simulink library "experiment_lib"  (Simulink 7.1)
values from neighbouring files (symbols this model uses):
  denPQ = [1 -0.999371878799]    [Pau_Pol_6_Nodes_4_Perd_0_TxRate_0.01.mat]
  LL = [0.000782892151765 0.000588394714514 0.000709966836418 0.00082261967749]    [Pau_Pol_6_Nodes_4_Perd_0_TxRate_0.01.mat]    (also in llencadora_sim.m = minLL+(maxLL-minLL)*rand(1,num_loads))
  Lline = [1.0827664502e-05 1.06430432216e-05 1.0255354423e-05 1.05299829153e-05]    [Pau_Pol_6_Nodes_4_Perd_0_TxRate_0.01.mat]    (also in llencadora_sim.m = minLline+(maxLline-minLline)*rand(1,num_lines))
  Lv = 1.28e-05    [Pau_Pol_6_Nodes_4_Perd_0_TxRate_0.01.mat]    (also in llencadora_sim.m = Lvm(nodes); processor.m = data.Lv)
  m = 1e-05    [Pau_Pol_6_Nodes_4_Perd_0_TxRate_0.01.mat]    (also in llencadora_sim.m; processor.m = data.m)
  mp = 5e-07    [Pau_Pol_6_Nodes_4_Perd_0_TxRate_0.01.mat]    (also in llencadora_sim.m = mpm(nodes); processor.m = data.mp)
  n = 0.0001    [Pau_Pol_6_Nodes_4_Perd_0_TxRate_0.01.mat]    (also in llencadora_sim.m; processor.m = data.n)
  numPQ = [0.000314060600312 0.000314060600312]    [Pau_Pol_6_Nodes_4_Perd_0_TxRate_0.01.mat]
  RL = [0.345490722943 0.282580500651 0.390474448437 0.324054882207]    [Pau_Pol_6_Nodes_4_Perd_0_TxRate_0.01.mat]    (also in llencadora_sim.m = minRL+(maxRL-minRL)*rand(1,num_loads))
  Rline = [0.00149363403679 0.00820725625814 0.00655593060546 0.00272568602759]    [Pau_Pol_6_Nodes_4_Perd_0_TxRate_0.01.mat]    (also in llencadora_sim.m = minRline+(maxRline-minRline)*rand(1,num_lines))
  tr = 0.01    [Pau_Pol_6_Nodes_4_Perd_0_TxRate_0.01.mat]    (also in llencadora_sim.m = 10)
  ts = 0.0001    [Pau_Pol_6_Nodes_4_Perd_0_TxRate_0.01.mat]    (also in dintegral_w_code.m; llencadora_sim.m; processor.m = data.ts)
  Vn = 325.269119346    [Pau_Pol_6_Nodes_4_Perd_0_TxRate_0.01.mat]    (also in llencadora_sim.m = 230*sqrt(2); processor.m = data.Vn)
  wo = 314.159265359    [Pau_Pol_6_Nodes_4_Perd_0_TxRate_0.01.mat]    (also in llencadora_sim.m; processor.m = data.wo)
undefined symbols (not defined in the file or in its folder): CL
libraries: powerlib x24, truetime x2
settings Model: Creator=SEPIC  LastModifiedBy=SEPIC

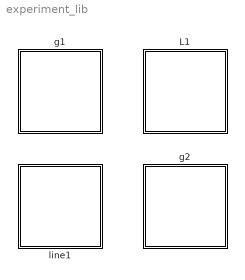
== system experiment_lib ==
  L1 : Subsystem  Orientation=down  mask{a=1}
      mask Display: disp(['Load' num2str(a)])
  g1 : Subsystem  Orientation=down  mask{a=1}
      mask Display: disp(['Gen' num2str(a)]);port_label('PMC',1,'a')
  g2 : Subsystem  Orientation=down  mask{a=1}
      mask Display: disp(['GenCom' num2str(a)]);port_label('PMC',1,'a')
  line1 : Subsystem  Orientation=left  mask{a=1}
      mask Display: disp(['Line' num2str(a)]);

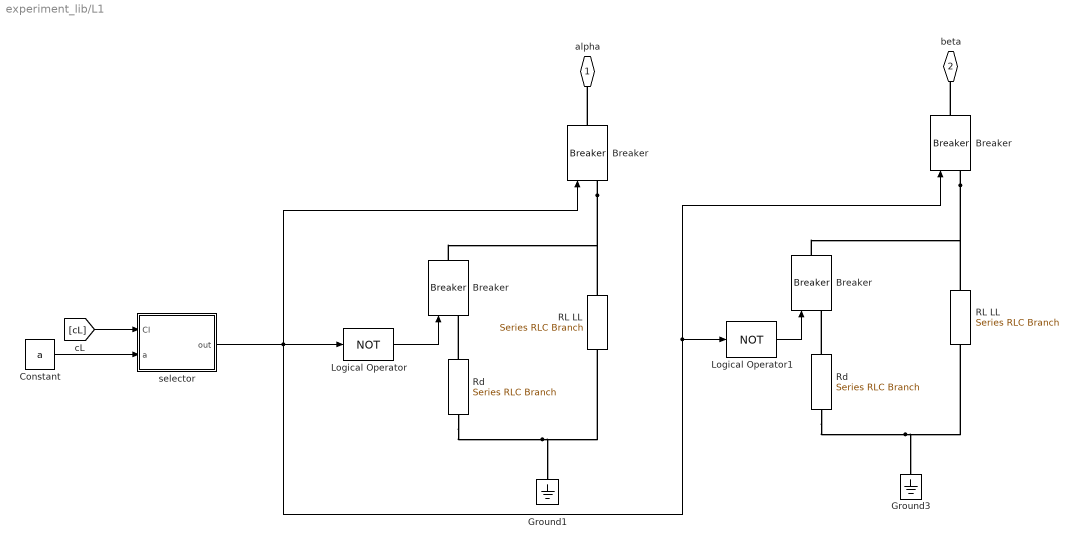
== system experiment_lib/L1 ==
  "  Rd" : powerlib/Elements/Series RLC Branch  Orientation=down  DialogController=POWERSYS.PowerSysDialog  PhysicalDomain=powersysdomain  SubClassName=unknown  LeftPortType=p1  RightPortType=p1  LConnTagsString=__new0  RConnTagsString=__new0  BranchType=R  Resistance=1  Inductance=1.0  SetiL0=off  InitialCurrent=0  Capacitance=CL  Setx0=off  InitialVoltage=0  Measurements=None
  "  Rd  " : powerlib/Elements/Series RLC Branch  Orientation=down  DialogController=POWERSYS.PowerSysDialog  PhysicalDomain=powersysdomain  SubClassName=unknown  LeftPortType=p1  RightPortType=p1  LConnTagsString=__new0  RConnTagsString=__new0  BranchType=R  Resistance=1  Inductance=1.0  SetiL0=off  InitialCurrent=0  Capacitance=CL  Setx0=off  InitialVoltage=0  Measurements=None
  Breaker : powerlib/Elements/Breaker  Orientation=up  DialogController=POWERSYS.PowerSysDialog  SystemSampleTime=-1  BreakerResistance=10e-6  InitialState=0  SnubberResistance=1e6  SnubberCapacitance=inf  SwitchingTimes="[ 1/60  5/60 ]"  External=on  Measurements=None  MoreParameters=off  NoBreakLoop=off
  "Breaker " : powerlib/Elements/Breaker  Orientation=up  DialogController=POWERSYS.PowerSysDialog  SystemSampleTime=-1  BreakerResistance=10e-6  InitialState=0  SnubberResistance=1e6  SnubberCapacitance=inf  SwitchingTimes="[ 1/60  5/60 ]"  External=on  Measurements=None  MoreParameters=off  NoBreakLoop=off
  "Breaker   " : powerlib/Elements/Breaker  Orientation=up  DialogController=POWERSYS.PowerSysDialog  SystemSampleTime=-1  BreakerResistance=10e-6  InitialState=0  SnubberResistance=1e6  SnubberCapacitance=inf  SwitchingTimes="[ 1/60  5/60 ]"  External=on  Measurements=None  MoreParameters=off  NoBreakLoop=off
  "Breaker      " : powerlib/Elements/Breaker  Orientation=up  DialogController=POWERSYS.PowerSysDialog  SystemSampleTime=-1  BreakerResistance=10e-6  InitialState=0  SnubberResistance=1e6  SnubberCapacitance=inf  SwitchingTimes="[ 1/60  5/60 ]"  External=on  Measurements=None  MoreParameters=off  NoBreakLoop=off
  Constant : Constant  Value=a  OutDataType=sfix(16)  OutScaling=2^0
  Ground1 : powerlib/Elements/Ground  Orientation=down  DialogController=POWERSYS.PowerSysDialog  PhysicalDomain=powersysdomain  SubClassName=unknown  LeftPortType=p1  RightPortType=p1  LConnTagsString=a
  Ground3 : powerlib/Elements/Ground  Orientation=down  DialogController=POWERSYS.PowerSysDialog  PhysicalDomain=powersysdomain  SubClassName=unknown  LeftPortType=p1  RightPortType=p1  LConnTagsString=a
  Logical Operator : Logic  Operator=NOT  AllPortsSameDT=off  OutDataTypeMode=boolean  OutDataTypeStr=boolean
  Logical Operator1 : Logic  Operator=NOT  AllPortsSameDT=off  OutDataTypeMode=boolean  OutDataTypeStr=boolean
  RL LL : powerlib/Elements/Series RLC Branch  Orientation=down  DialogController=POWERSYS.PowerSysDialog  PhysicalDomain=powersysdomain  SubClassName=unknown  LeftPortType=p1  RightPortType=p1  LConnTagsString=__new0  RConnTagsString=__new0  BranchType=RL  Resistance=RL(a)  Inductance=LL(a)  SetiL0=off  InitialCurrent=0  Capacitance=CL  Setx0=off  InitialVoltage=0  Measurements=None
  "RL LL   " : powerlib/Elements/Series RLC Branch  Orientation=down  DialogController=POWERSYS.PowerSysDialog  PhysicalDomain=powersysdomain  SubClassName=unknown  LeftPortType=p1  RightPortType=p1  LConnTagsString=__new0  RConnTagsString=__new0  BranchType=RL  Resistance=RL(a)  Inductance=LL(a)  SetiL0=off  InitialCurrent=0  Capacitance=CL  Setx0=off  InitialVoltage=0  Measurements=None
  selector : Stateflow chart  TreatAsAtomicUnit=on
  "alpha " : PMIOPort  Orientation=down  Port=1  Side=Left
  beta : PMIOPort  Orientation=down  Port=2  Side=Left
  wires:
  Logical Operator/1 -> Breaker/1
  selector/1(out) -> Logical Operator/1, "Breaker      "/1, Logical Operator1/1, "Breaker   "/1
  Logical Operator1/1 -> "Breaker "/1
  [cL] -> selector/1(Cl)
  Constant/1 -> selector/2(a)
  connections:
  "Breaker      "/LConn1 -- Breaker/RConn1 -- RL LL/LConn1
  "  Rd"/RConn1 -- RL LL/RConn1 -- Ground1/LConn1
  "  Rd"/LConn1 -- Breaker/LConn1
  "Breaker      "/RConn1 -- "alpha "/RConn1
  "Breaker   "/LConn1 -- "RL LL   "/LConn1 -- "Breaker "/RConn1
  "  Rd  "/RConn1 -- Ground3/LConn1 -- "RL LL   "/RConn1
  "  Rd  "/LConn1 -- "Breaker "/LConn1
  "Breaker   "/RConn1 -- beta/RConn1

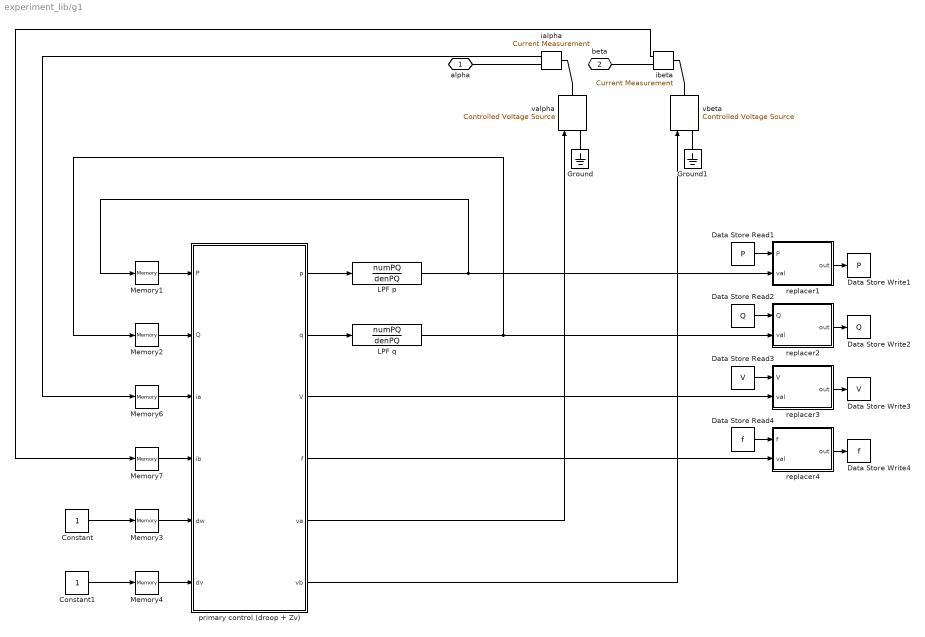
== system experiment_lib/g1 ==
  Constant : Constant  OutDataType=sfix(16)  OutScaling=2^0
  Constant1 : Constant  OutDataType=sfix(16)  OutScaling=2^0
  Data Store Read1 : DataStoreRead  DataStoreName=P  SampleTime=0
  Data Store Read2 : DataStoreRead  DataStoreName=Q  SampleTime=0
  Data Store Read3 : DataStoreRead  DataStoreName=V  SampleTime=0
  Data Store Read4 : DataStoreRead  DataStoreName=f  SampleTime=0
  Data Store Write1 : DataStoreWrite  DataStoreName=P  SampleTime=-1
  Data Store Write2 : DataStoreWrite  DataStoreName=Q  SampleTime=-1
  Data Store Write3 : DataStoreWrite  DataStoreName=V  SampleTime=-1
  Data Store Write4 : DataStoreWrite  DataStoreName=f  SampleTime=-1
  Ground : powerlib/Elements/Ground  Orientation=down  DialogController=POWERSYS.PowerSysDialog  PhysicalDomain=powersysdomain  SubClassName=unknown  LeftPortType=p1  RightPortType=p1  LConnTagsString=a
  Ground1 : powerlib/Elements/Ground  Orientation=down  DialogController=POWERSYS.PowerSysDialog  PhysicalDomain=powersysdomain  SubClassName=unknown  LeftPortType=p1  RightPortType=p1  LConnTagsString=a
  LPF p : DiscreteTransferFcn  Numerator=numPQ  Denominator=denPQ  SampleTime=ts
  LPF q : DiscreteTransferFcn  Numerator=numPQ  Denominator=denPQ  SampleTime=ts
  Memory{1..4,6..7} (6 alike) : Memory
  ialpha : powerlib/Measurements/Current Measurement  Orientation=left  DialogController=POWERSYS.PowerSysDialog  SystemSampleTime=-1  PhasorSimulation=off  OutputType=Complex  PSBequivalent=0
  ibeta : powerlib/Measurements/Current Measurement  Orientation=left  DialogController=POWERSYS.PowerSysDialog  SystemSampleTime=-1  PhasorSimulation=off  OutputType=Complex  PSBequivalent=0
  primary control (droop + Zv) : Stateflow chart  TreatAsAtomicUnit=on
  replacer1 : Stateflow chart  TreatAsAtomicUnit=on
  replacer2 : Stateflow chart  TreatAsAtomicUnit=on
  replacer3 : Stateflow chart  TreatAsAtomicUnit=on
  replacer4 : Stateflow chart  TreatAsAtomicUnit=on
  valpha : powerlib/Electrical Sources/Controlled Voltage Source  Orientation=up  DialogController=POWERSYS.PowerSysDialog  SystemSampleTime=-1  Initialize=on  Source_Type=AC  Amplitude=0  Phase=0  Frequency=0  Measurements=None
  vbeta : powerlib/Electrical Sources/Controlled Voltage Source  Orientation=up  DialogController=POWERSYS.PowerSysDialog  SystemSampleTime=-1  Initialize=on  Source_Type=AC  Amplitude=0  Phase=0  Frequency=0  Measurements=None
  alpha : PMIOPort  Port=1  Side=Left
  beta : PMIOPort  Port=2  Side=Left
  wires:
  ibeta/1 -> Memory7/1
  ialpha/1 -> Memory6/1
  LPF p/1 -> Memory1/1, replacer1/2(val)
  LPF q/1 -> Memory2/1, replacer2/2(val)
  primary control (droop + Zv)/1(p) -> LPF p/1
  primary control (droop + Zv)/2(q) -> LPF q/1
  primary control (droop + Zv)/4(f) -> replacer4/2(val)
  primary control (droop + Zv)/3(V) -> replacer3/2(val)
  Memory6/1 -> primary control (droop + Zv)/3(ia)
  Memory7/1 -> primary control (droop + Zv)/4(ib)
  Memory1/1 -> primary control (droop + Zv)/1(P)
  Memory2/1 -> primary control (droop + Zv)/2(Q)
  Memory3/1 -> primary control (droop + Zv)/5(dw)
  Memory4/1 -> primary control (droop + Zv)/6(dv)
  primary control (droop + Zv)/5(va) -> valpha/1
  primary control (droop + Zv)/6(vb) -> vbeta/1
  Constant/1 -> Memory3/1
  Constant1/1 -> Memory4/1
  replacer1/1(out) -> Data Store Write1/1
  replacer2/1(out) -> Data Store Write2/1
  Data Store Read2/1 -> replacer2/1(Q)
  replacer3/1(out) -> Data Store Write3/1
  Data Store Read3/1 -> replacer3/1(V)
  Data Store Read1/1 -> replacer1/1(P)
  replacer4/1(out) -> Data Store Write4/1
  Data Store Read4/1 -> replacer4/1(f)
  connections:
  Ground1/LConn1 -- vbeta/LConn1
  valpha/RConn1 -- ialpha/LConn1
  beta/RConn1 -- ibeta/RConn1
  vbeta/RConn1 -- ibeta/LConn1
  Ground/LConn1 -- valpha/LConn1
  alpha/RConn1 -- ialpha/RConn1

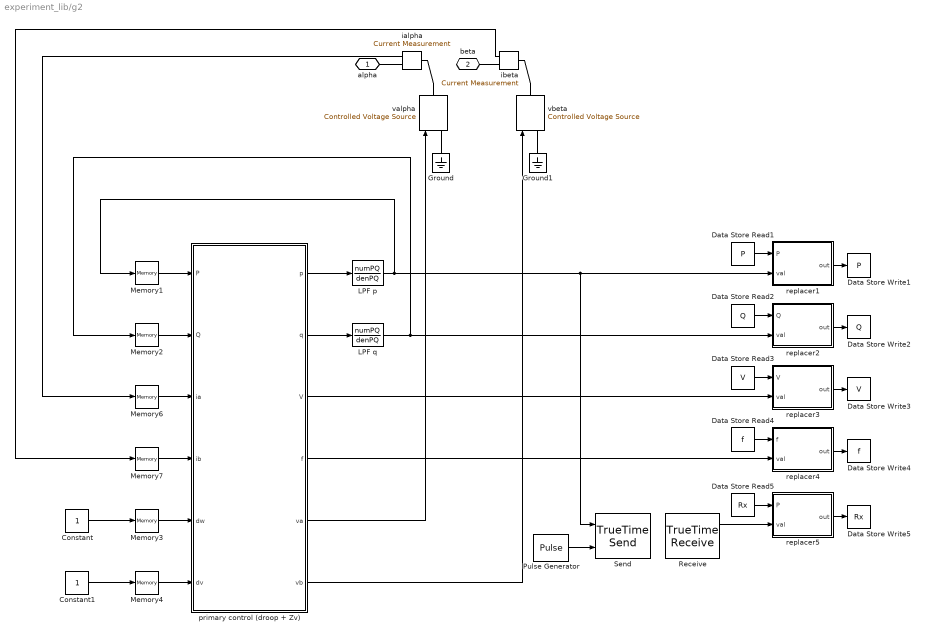
== system experiment_lib/g2 ==
  Constant : Constant  OutDataType=sfix(16)  OutScaling=2^0
  Constant1 : Constant  OutDataType=sfix(16)  OutScaling=2^0
  Data Store Read1 : DataStoreRead  DataStoreName=P  SampleTime=0
  Data Store Read2 : DataStoreRead  DataStoreName=Q  SampleTime=0
  Data Store Read3 : DataStoreRead  DataStoreName=V  SampleTime=0
  Data Store Read4 : DataStoreRead  DataStoreName=f  SampleTime=0
  Data Store Read5 : DataStoreRead  DataStoreName=Rx  SampleTime=0
  Data Store Write1 : DataStoreWrite  DataStoreName=P  SampleTime=-1
  Data Store Write2 : DataStoreWrite  DataStoreName=Q  SampleTime=-1
  Data Store Write3 : DataStoreWrite  DataStoreName=V  SampleTime=-1
  Data Store Write4 : DataStoreWrite  DataStoreName=f  SampleTime=-1
  Data Store Write5 : DataStoreWrite  DataStoreName=Rx  SampleTime=-1
  Ground : powerlib/Elements/Ground  Orientation=down  DialogController=POWERSYS.PowerSysDialog  PhysicalDomain=powersysdomain  SubClassName=unknown  LeftPortType=p1  RightPortType=p1  LConnTagsString=a
  Ground1 : powerlib/Elements/Ground  Orientation=down  DialogController=POWERSYS.PowerSysDialog  PhysicalDomain=powersysdomain  SubClassName=unknown  LeftPortType=p1  RightPortType=p1  LConnTagsString=a
  LPF p : DiscreteTransferFcn  Numerator=numPQ  Denominator=denPQ  SampleTime=ts
  LPF q : DiscreteTransferFcn  Numerator=numPQ  Denominator=denPQ  SampleTime=ts
  Memory{1..4,6..7} (6 alike) : Memory
  Pulse Generator : DiscretePulseGenerator  PulseType=Time based  Period=tr  PulseWidth=50
  Receive : truetime/TrueTime Receive  SystemSampleTime=-1  nwnbr=1  receiver=a  outdim=1  triggeroutput=off  senderoutput=on  lengthoutput=off  priorityoutput=off  timestampoutput=off  signalpoweroutput=off  msgIDoutput=off
  Send : truetime/TrueTime Send  SystemSampleTime=-1  trigger=rising  nwnbr=1  sender=a  indim=1  recsource=internal  receiver=0  lengthsource=internal  length=80  priosource=internal  prio=2  msgIDsource=internal  msgID=0  dynamicSegment=dynamic
  ialpha : powerlib/Measurements/Current Measurement  Orientation=left  DialogController=POWERSYS.PowerSysDialog  SystemSampleTime=-1  PhasorSimulation=off  OutputType=Complex  PSBequivalent=0
  ibeta : powerlib/Measurements/Current Measurement  Orientation=left  DialogController=POWERSYS.PowerSysDialog  SystemSampleTime=-1  PhasorSimulation=off  OutputType=Complex  PSBequivalent=0
  primary control (droop + Zv) : Stateflow chart  TreatAsAtomicUnit=on
  replacer1 : Stateflow chart  TreatAsAtomicUnit=on
  replacer2 : Stateflow chart  TreatAsAtomicUnit=on
  replacer3 : Stateflow chart  TreatAsAtomicUnit=on
  replacer4 : Stateflow chart  TreatAsAtomicUnit=on
  replacer5 : Stateflow chart  TreatAsAtomicUnit=on
  valpha : powerlib/Electrical Sources/Controlled Voltage Source  Orientation=up  DialogController=POWERSYS.PowerSysDialog  SystemSampleTime=-1  Initialize=on  Source_Type=AC  Amplitude=0  Phase=0  Frequency=0  Measurements=None
  vbeta : powerlib/Electrical Sources/Controlled Voltage Source  Orientation=up  DialogController=POWERSYS.PowerSysDialog  SystemSampleTime=-1  Initialize=on  Source_Type=AC  Amplitude=0  Phase=0  Frequency=0  Measurements=None
  alpha : PMIOPort  Port=1  Side=Left
  beta : PMIOPort  Port=2  Side=Left
  wires:
  Data Store Read4/1 -> replacer4/1(f)
  replacer4/1(out) -> Data Store Write4/1
  Data Store Read1/1 -> replacer1/1(P)
  Data Store Read3/1 -> replacer3/1(V)
  replacer3/1(out) -> Data Store Write3/1
  Data Store Read2/1 -> replacer2/1(Q)
  replacer2/1(out) -> Data Store Write2/1
  replacer1/1(out) -> Data Store Write1/1
  Constant1/1 -> Memory4/1
  Constant/1 -> Memory3/1
  primary control (droop + Zv)/6(vb) -> vbeta/1
  primary control (droop + Zv)/5(va) -> valpha/1
  Memory4/1 -> primary control (droop + Zv)/6(dv)
  Memory3/1 -> primary control (droop + Zv)/5(dw)
  Memory2/1 -> primary control (droop + Zv)/2(Q)
  Memory1/1 -> primary control (droop + Zv)/1(P)
  Memory7/1 -> primary control (droop + Zv)/4(ib)
  Memory6/1 -> primary control (droop + Zv)/3(ia)
  primary control (droop + Zv)/3(V) -> replacer3/2(val)
  primary control (droop + Zv)/4(f) -> replacer4/2(val)
  primary control (droop + Zv)/2(q) -> LPF q/1
  primary control (droop + Zv)/1(p) -> LPF p/1
  LPF q/1 -> replacer2/2(val), Memory2/1
  LPF p/1 -> Memory1/1, replacer1/2(val), Send/1
  ialpha/1 -> Memory6/1
  ibeta/1 -> Memory7/1
  Pulse Generator/1 -> Send/2
  Data Store Read5/1 -> replacer5/1(P)
  replacer5/1(out) -> Data Store Write5/1
  Receive/1 -> replacer5/2(val)
  connections:
  alpha/RConn1 -- ialpha/RConn1
  Ground/LConn1 -- valpha/LConn1
  vbeta/RConn1 -- ibeta/LConn1
  beta/RConn1 -- ibeta/RConn1
  valpha/RConn1 -- ialpha/LConn1
  Ground1/LConn1 -- vbeta/LConn1

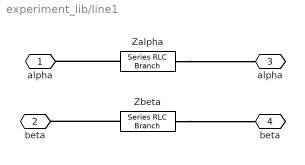
== system experiment_lib/line1 ==
  Zalpha : powerlib/Elements/Series RLC Branch  Orientation=left  DialogController=POWERSYS.PowerSysDialog  PhysicalDomain=powersysdomain  SubClassName=unknown  LeftPortType=p1  RightPortType=p1  LConnTagsString=__new0  RConnTagsString=__new0  BranchType=RL  Resistance=Rline(a)  Inductance=Lline(a)  SetiL0=off  InitialCurrent=0  Capacitance=CL  Setx0=off  InitialVoltage=0  Measurements=None
  Zbeta : powerlib/Elements/Series RLC Branch  Orientation=left  DialogController=POWERSYS.PowerSysDialog  PhysicalDomain=powersysdomain  SubClassName=unknown  LeftPortType=p1  RightPortType=p1  LConnTagsString=__new0  RConnTagsString=__new0  BranchType=RL  Resistance=Rline(a)  Inductance=Lline(a)  SetiL0=off  InitialCurrent=0  Capacitance=CL  Setx0=off  InitialVoltage=0  Measurements=None
  alpha : PMIOPort  Port=1  Side=Left
  "beta " : PMIOPort  Port=2  Side=Left
  "alpha " : PMIOPort  Orientation=left  Port=3  Side=Right
  "beta   " : PMIOPort  Orientation=left  Port=4  Side=Right
  connections:
  Zbeta/RConn1 -- "beta "/RConn1
  Zbeta/LConn1 -- "beta   "/RConn1
  Zalpha/RConn1 -- alpha/RConn1
  Zalpha/LConn1 -- "alpha "/RConn1

== matlab function g1/replacer1 ==
  data: P input double; out output double; val input double; a parameter double
function out  = fcn2(P,val,a)
out=P;
out(a)=val;

== matlab function g1/replacer2 ==
  data: Q input double; out output double; val input double; a parameter double
function out  = fcn2(Q,val,a)
out=Q;
out(a)=val;

== matlab function g1/replacer3 ==
  data: V input double; out output double; val input double; a parameter double
function out  = fcn2(V,val,a)
out=V;
out(a)=val;

== matlab function L1/selector ==
  data: Cl input double; out output double; a input double
function out  = fcn2(Cl,a)
out=Cl(a);

== matlab function g1/replacer4 ==
  data: f input double; out output double; val input double; a parameter double
function out  = fcn2(f,val,a)
out=f;
out(a)=val;

== matlab function g2/primary control (droop + Zv) ==
  settings: updateMethod=DISCRETE  sampleTime=ts
  data: P input double; Q input double; ia input double size=1; p output double; q output double; ib input double; V output double; f output double; va output double; vb output double; dw input double; dv input double; Vn parameter double; wo parameter double; m parameter double; n parameter double; mp parameter double; Lv parameter double; ts parameter double
function [p,q,V,f,va,vb]  = fcn2(P,Q,ia,ib,dw,dv,Vn,wo,m,n,mp,Lv,ts)

persistent t; if isempty(t); t=0; end; % ta = float('double')

t=t+ts; ph=(wo+dw-m*P)*t-mp*P; if ph>(2*pi) t=((ph-2*pi)+mp*P)/(wo+dw-m*P); end;
va=(Vn+dv-n*Q)*sin(ph); vb=-(Vn+dv-n*Q)*cos(ph);
va=va+Lv*wo*ib; vb=vb-Lv*wo*ia;

p=(3/2)*(va*ia+vb*ib); q=(3/2)*(-va*ib+vb*ia);
V=sqrt(va^2+vb^2); f=(wo+dw-m*P)/(2*pi);

== matlab function g2/replacer1 ==
  data: P input double; out output double; val input double; a parameter double
function out  = fcn2(P,val,a)
out=P;
out(a)=val;

== matlab function g1/primary control (droop + Zv) ==
  settings: updateMethod=DISCRETE  sampleTime=ts
  data: P input double; Q input double; ia input double size=1; p output double; q output double; ib input double; V output double; f output double; va output double; vb output double; dw input double; dv input double; Vn parameter double; wo parameter double; m parameter double; n parameter double; mp parameter double; Lv parameter double; ts parameter double
function [p,q,V,f,va,vb]  = fcn2(P,Q,ia,ib,dw,dv,Vn,wo,m,n,mp,Lv,ts)

persistent t; if isempty(t); t=0; end; % ta = float('double')

t=t+ts; ph=(wo+dw-m*P)*t-mp*P; if ph>(2*pi) t=((ph-2*pi)+mp*P)/(wo+dw-m*P); end;
va=(Vn+dv-n*Q)*sin(ph); vb=-(Vn+dv-n*Q)*cos(ph);
va=va+Lv*wo*ib; vb=vb-Lv*wo*ia;

p=(3/2)*(va*ia+vb*ib); q=(3/2)*(-va*ib+vb*ia);
V=sqrt(va^2+vb^2); f=(wo+dw-m*P)/(2*pi);

== matlab function g2/replacer2 ==
  data: Q input double; out output double; val input double; a parameter double
function out  = fcn2(Q,val,a)
out=Q;
out(a)=val;

== matlab function g2/replacer3 ==
  data: V input double; out output double; val input double; a parameter double
function out  = fcn2(V,val,a)
out=V;
out(a)=val;

== matlab function g2/replacer4 ==
  data: f input double; out output double; val input double; a parameter double
function out  = fcn2(f,val,a)
out=f;
out(a)=val;

== matlab function g2/replacer5 ==
  data: P input double; out output double; val input double; a parameter double
function out  = fcn2(P,val,a)
out=P;
out(a)=val;
